simulink model "untitled"  (R2018a)
settings: Solver=VariableStepAuto  StartTime=0.0  StopTime=10.0  RelTol=1e-3
model workspace (MAT data in the model file):
  p0 = 0
  p1 = 0
  p2 = 0
  p3 = 0
settings Model: Creator=adiravishankara  LastModifiedBy=adiravishankara

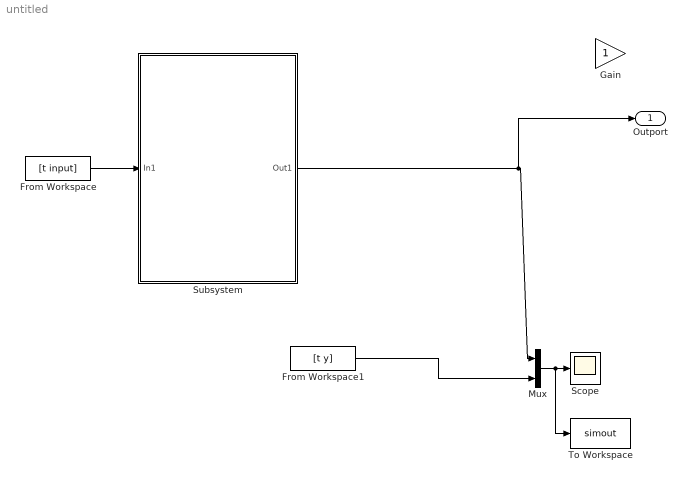
== system untitled ==
  From Workspace : FromWorkspace  VariableName=[t input]  SampleTime=0
  From Workspace1 : FromWorkspace  VariableName=[t y]  SampleTime=0
  Gain : Gain
  Mux : Mux  Inputs=2
  Scope : Scope
  Subsystem : Subsystem
  To Workspace : ToWorkspace  VariableName=simout  SaveFormat=Timeseries  SampleTime=-1
  Outport : Outport
  wires:
  Subsystem/1(Out1) -> Outport/1, Mux/1
  Mux/1 -> To Workspace/1, Scope/1
  From Workspace1/1 -> Mux/2
  From Workspace/1 -> Subsystem/1(In1)

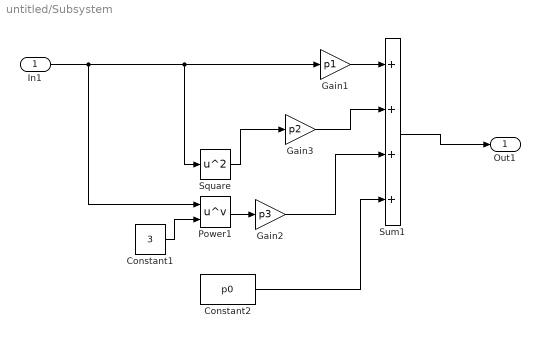
== system untitled/Subsystem ==
  In1 : Inport
  Constant1 : Constant  Value=3
  Constant2 : Constant  Value=p0
  Gain1 : Gain  Gain=p1
  Gain2 : Gain  Gain=p3
  Gain3 : Gain  Gain=p2
  Power1 : Math  Operator=pow  SaturateOnIntegerOverflow=on
  Square : Math  Operator=square  SaturateOnIntegerOverflow=on
  Sum1 : Sum  Inputs=++++
  Out1 : Outport
  wires:
  Gain2/1 -> Sum1/3
  Constant1/1 -> Power1/2
  Gain1/1 -> Sum1/1
  Power1/1 -> Gain2/1
  In1/1 -> Power1/1, Square/1, Gain1/1
  Sum1/1 -> Out1/1
  Constant2/1 -> Sum1/4
  Square/1 -> Gain3/1
  Gain3/1 -> Sum1/2
